simulink model "STEVE_Simulation_6DOF"  (R2025b)
settings: Solver=ode45  StartTime=0  StopTime=60  FixedStep=0.0001  MaxStep=0.0001  RelTol=1e-3
model workspace (MAT data in the model file):
  op_trim1 : opcond.OperatingReport (value not decoded)
undefined symbols (not defined in the file): Actuators, AeroData, C_inner_maxQ_d_Ki, C_inner_maxQ_d_Kp, C_outer_maxQ_d_Ki, C_outer_maxQ_d_Kp, F, launchpad_alt, Light, MIL, PrelookupData, Ref_Area, rocket_length, timeStep, Ts_inner, Ts_outer, warm_up_time, wn_ramp
libraries: simulink_extras x23, simulink x7, slpidlib x5, aerolibwind2 x3, aerolibconvert2 x3, aerolibasang x2, aerolibactuator x2, aerolibatmos2 x1
(part 2 of 2)

== system STEVE_Simulation_6DOF/STeVe System Model/Subsystem/Classical Upgraded/Cascade PID Controller1 ==
  pitch rate : Inport
  pitch : Inport  Port=2
  pitch_setpoint : Inport  Port=3
  Add : Sum  Inputs=-+
  Add1 : Sum  Inputs=-+
  Pitch Controller : slpidlib/PID Controller  Controller=PI  Form=Parallel  TimeDomain=Discrete-time  UseExternalTs=off  SampleTime=Ts_outer  IntegratorMethod=Forward Euler  FilterMethod=Forward Euler  ControllerParametersSource=internal  P=C_outer_maxQ_d_Kp  I=C_outer_maxQ_d_Ki  UseKiTs=off  D=0.164283893804061  UseExternalDerivativeSource=off  N=4651.32243718652  UseFilter=on  TunerSelectOption=Transfer Function Based (PID Tuner App)  InitialConditionSource=internal  InitialConditionForIntegrator=0  InitialConditionForFilter=0  DifferentiatorICPrevScaledInput=0  ExternalReset=none  TrackingMode=off  Kt=1  LimitOutput=off  SatLimitsSource=internal  UpperSaturationLimit=inf  LowerSaturationLimit=-inf  LinearizeAsGain=on  AntiWindupMode=none  Kb=1  LimitIntegrator=off  UpperIntegratorSaturationLimit=inf  LowerIntegratorSaturationLimit=-inf  POutMin=[]  POutMax=[]  IOutMin=[]  IOutMax=[]  DOutMin=[]  DOutMax=[]  NOutMin=[]  NOutMax=[]  SumOutMin=[]  SumOutMax=[]  SaturationOutMin=[]  SaturationOutMax=[]  PParamMin=[]  PParamMax=[]  IParamMin=[]  IParamMax=[]  DParamMin=[]  DParamMax=[]  NParamMin=[]  NParamMax=[]  KbParamMin=[]  KbParamMax=[]  KtParamMin=[]  KtParamMax=[]  KbOutMin=[]  KbOutMax=[]  KtOutMin=[]  KtOutMax=[]  IntegratorOutMin=[]  IntegratorOutMax=[]  FilterOutMin=[]  FilterOutMax=[]  SumI1OutMin=[]  SumI1OutMax=[]  SumI2OutMin=[]  SumI2OutMax=[]  SumI3OutMin=[]  SumI3OutMax=[]  SumI4OutMin=[]  SumI4OutMax=[]  SumDOutMin=[]  SumDOutMax=[]  DifferentiatorOutMin=[]  DifferentiatorOutMax=[]  FilterDiffOutCoefMin=[]  FilterDiffOutCoefMax=[]  ReciprocalOutMin=[]  ReciprocalOutMax=[]  SumDenOutMin=[]  SumDenOutMax=[]  SumNumOutMin=[]  SumNumOutMax=[]  DivideOutMin=[]  DivideOutMax=[]  UdiffTsProdOutMin=[]  UdiffTsProdOutMax=[]  NTsProdOutMin=[]  NTsProdOutMax=[]  UintegralTsProdOutMin=[]  UintegralTsProdOutMax=[]  UngainTsProdOutMin=[]  UngainTsProdOutMax=[]  ClampingZeroOutDataTypeStr=Inherit: Inherit via back propagation  ClampingZeroOutMin=[]  ClampingZeroOutMax=[]  FilterDenConstantOutDataTypeStr=Inherit: Inherit via back propagation  FilterDenConstantOutMin=[]  FilterDenConstantOutMax=[]  PCopyOutDataTypeStr=Inherit: Inherit via back propagation  PCopyOutMin=[]  PCopyOutMax=[]  NCopyOutDataTypeStr=Inherit: Inherit via back propagation  NCopyOutMin=[]  NCopyOutMax=[]  IntegratorContinuousStateAttributes=''  IntegratorStateMustResolveToSignalObject=off  IntegratorRTWStateStorageClass=Auto  FilterContinuousStateAttributes=''  FilterStateMustResolveToSignalObject=off  FilterRTWStateStorageClass=Auto  ParallelPVariant=InternalParameters  IdealPVariant=Disabled  IVariant=InternalParameters  DVariant=Disabled  IntegratorVariant=Discrete  SatVariant=Disabled  AWVariant=Passthrough  PCopyVariant=Disabled  TRVariant=Disabled  FdbkBlocksVariant=Forward  IdealPFdbkVariant=Disabled  SatFdbkVariant=Disabled  DerivativeFilterVariant=Disabled  NVariant=Disabled  NCopyVariant=Disabled_SignalSpec  FilterICVariant=Disabled  IntegratorICVariant=InternalICs  ExternalResetVariant=Disabled  TRSumVariant=Passthrough  SumFdbkVariant=Disabled  SumVariant=Sum_PI  TsampFilterVariant=InternalTs  TsampNgainVariant=Passthrough  TsampIntegralVariant=Disabled_SignalSpec  ExternalSaturationOutDataTypeStr=Inherit: Same as second input  DerivativeSourceVariant=Disabled  PreIntVariant=InternalPreInt
  Pitch Rate Controller : slpidlib/PID Controller  Controller=PI  Form=Parallel  TimeDomain=Discrete-time  UseExternalTs=off  SampleTime=Ts_inner  IntegratorMethod=Forward Euler  FilterMethod=Forward Euler  ControllerParametersSource=internal  P=C_inner_maxQ_d_Kp  I=C_inner_maxQ_d_Ki  UseKiTs=off  D=0.164283893804061  UseExternalDerivativeSource=off  N=4651.32243718652  UseFilter=on  TunerSelectOption=Transfer Function Based (PID Tuner App)  InitialConditionSource=internal  InitialConditionForIntegrator=0  InitialConditionForFilter=0  DifferentiatorICPrevScaledInput=0  ExternalReset=none  TrackingMode=off  Kt=1  LimitOutput=off  SatLimitsSource=internal  UpperSaturationLimit=inf  LowerSaturationLimit=-inf  LinearizeAsGain=on  AntiWindupMode=none  Kb=1  LimitIntegrator=off  UpperIntegratorSaturationLimit=inf  LowerIntegratorSaturationLimit=-inf  POutMin=[]  POutMax=[]  IOutMin=[]  IOutMax=[]  DOutMin=[]  DOutMax=[]  NOutMin=[]  NOutMax=[]  SumOutMin=[]  SumOutMax=[]  SaturationOutMin=[]  SaturationOutMax=[]  PParamMin=[]  PParamMax=[]  IParamMin=[]  IParamMax=[]  DParamMin=[]  DParamMax=[]  NParamMin=[]  NParamMax=[]  KbParamMin=[]  KbParamMax=[]  KtParamMin=[]  KtParamMax=[]  KbOutMin=[]  KbOutMax=[]  KtOutMin=[]  KtOutMax=[]  IntegratorOutMin=[]  IntegratorOutMax=[]  FilterOutMin=[]  FilterOutMax=[]  SumI1OutMin=[]  SumI1OutMax=[]  SumI2OutMin=[]  SumI2OutMax=[]  SumI3OutMin=[]  SumI3OutMax=[]  SumI4OutMin=[]  SumI4OutMax=[]  SumDOutMin=[]  SumDOutMax=[]  DifferentiatorOutMin=[]  DifferentiatorOutMax=[]  FilterDiffOutCoefMin=[]  FilterDiffOutCoefMax=[]  ReciprocalOutMin=[]  ReciprocalOutMax=[]  SumDenOutMin=[]  SumDenOutMax=[]  SumNumOutMin=[]  SumNumOutMax=[]  DivideOutMin=[]  DivideOutMax=[]  UdiffTsProdOutMin=[]  UdiffTsProdOutMax=[]  NTsProdOutMin=[]  NTsProdOutMax=[]  UintegralTsProdOutMin=[]  UintegralTsProdOutMax=[]  UngainTsProdOutMin=[]  UngainTsProdOutMax=[]  ClampingZeroOutDataTypeStr=Inherit: Inherit via back propagation  ClampingZeroOutMin=[]  ClampingZeroOutMax=[]  FilterDenConstantOutDataTypeStr=Inherit: Inherit via back propagation  FilterDenConstantOutMin=[]  FilterDenConstantOutMax=[]  PCopyOutDataTypeStr=Inherit: Inherit via back propagation  PCopyOutMin=[]  PCopyOutMax=[]  NCopyOutDataTypeStr=Inherit: Inherit via back propagation  NCopyOutMin=[]  NCopyOutMax=[]  IntegratorContinuousStateAttributes=''  IntegratorStateMustResolveToSignalObject=off  IntegratorRTWStateStorageClass=Auto  FilterContinuousStateAttributes=''  FilterStateMustResolveToSignalObject=off  FilterRTWStateStorageClass=Auto  ParallelPVariant=InternalParameters  IdealPVariant=Disabled  IVariant=InternalParameters  DVariant=Disabled  IntegratorVariant=Discrete  SatVariant=Disabled  AWVariant=Passthrough  PCopyVariant=Disabled  TRVariant=Disabled  FdbkBlocksVariant=Forward  IdealPFdbkVariant=Disabled  SatFdbkVariant=Disabled  DerivativeFilterVariant=Disabled  NVariant=Disabled  NCopyVariant=Disabled_SignalSpec  FilterICVariant=Disabled  IntegratorICVariant=InternalICs  ExternalResetVariant=Disabled  TRSumVariant=Passthrough  SumFdbkVariant=Disabled  SumVariant=Sum_PI  TsampFilterVariant=InternalTs  TsampNgainVariant=Passthrough  TsampIntegralVariant=Disabled_SignalSpec  ExternalSaturationOutDataTypeStr=Inherit: Same as second input  DerivativeSourceVariant=Disabled  PreIntVariant=InternalPreInt
  nozzle angle : Outport
  wires:
  pitch/1 -> Add/1
  pitch_setpoint/1 -> Add/2
  Add/1 -> Pitch Controller/1
  Add1/1 -> Pitch Rate Controller/1
  pitch rate/1 -> Add1/1
  Pitch Controller/1 -> Add1/2
  Pitch Rate Controller/1 -> nozzle angle/1

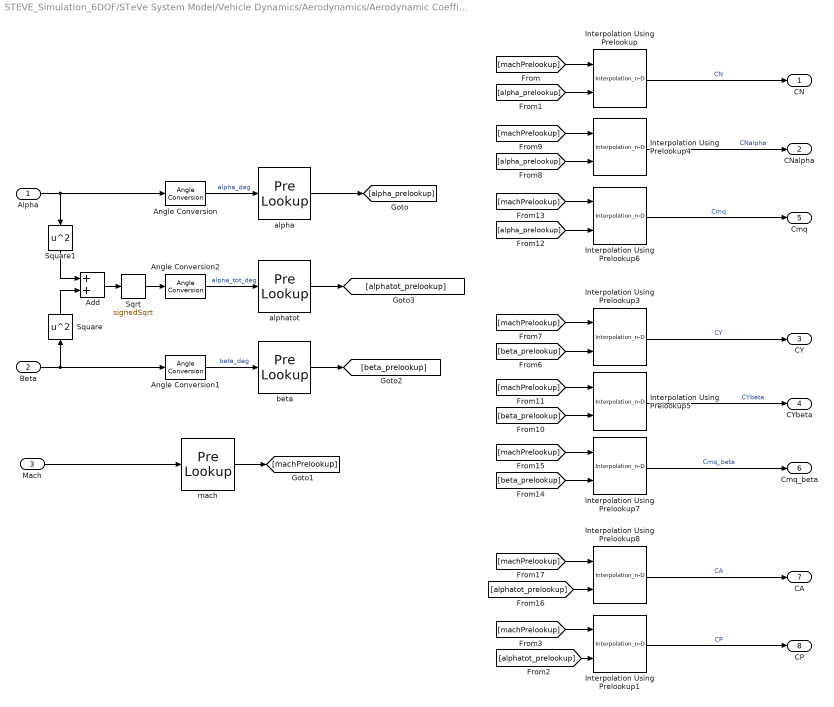
== system STEVE_Simulation_6DOF/STeVe System Model/Vehicle Dynamics/Aerodynamics/Aerodynamic Coefficients  ==
  Alpha : Inport
  Beta : Inport  Port=2
  Mach : Inport  Port=3
  Add : Sum
  Angle Conversion : aerolibconvert2/Angle Conversion  IU=rad  OU=deg
  Angle Conversion1 : aerolibconvert2/Angle Conversion  IU=rad  OU=deg
  Angle Conversion2 : aerolibconvert2/Angle Conversion  IU=rad  OU=deg
  Interpolation Using Prelookup : Interpolation_n-D  Table=AeroData.Tables.CN  RequireIndexFractionAsBus=on  InternalRulePriority=Speed
      settings: InputPortMap=u0,u1
  Interpolation Using Prelookup1 : Interpolation_n-D  Table=AeroData.Tables.CP  RequireIndexFractionAsBus=on  InternalRulePriority=Speed
      settings: InputPortMap=u0,u1
  Interpolation Using Prelookup3 : Interpolation_n-D  Table=AeroData.Tables.CY  RequireIndexFractionAsBus=on  InternalRulePriority=Speed
      settings: InputPortMap=u0,u1
  Interpolation Using Prelookup4 : Interpolation_n-D  Table=AeroData.Tables.CNalpha  RequireIndexFractionAsBus=on  InternalRulePriority=Speed
      settings: InputPortMap=u0,u1
  Interpolation Using Prelookup5 : Interpolation_n-D  Table=AeroData.Tables.CYbeta  RequireIndexFractionAsBus=on  InternalRulePriority=Speed
      settings: InputPortMap=u0,u1
  Interpolation Using Prelookup6 : Interpolation_n-D  Table=AeroData.Tables.Cmq  RequireIndexFractionAsBus=on  InternalRulePriority=Speed
      settings: InputPortMap=u0,u1
  Interpolation Using Prelookup7 : Interpolation_n-D  Table=AeroData.Tables.Cmq_beta  RequireIndexFractionAsBus=on  InternalRulePriority=Speed
      settings: InputPortMap=u0,u1
  Interpolation Using Prelookup8 : Interpolation_n-D  Table=AeroData.Tables.CA  RequireIndexFractionAsBus=on  InternalRulePriority=Speed
      settings: InputPortMap=u0,u1
  Sqrt : Sqrt  Operator=signedSqrt
  Square : Math  Operator=square
  Square1 : Math  Operator=square
  alpha : PreLookup  BreakpointsData=AeroData.Breakpoints.Alpha  OutputSelection=Index and fraction as bus  IndexSearchMethod=Evenly spaced points  UseLastBreakpoint=on
  alphatot : PreLookup  BreakpointsData=AeroData.Breakpoints.AlphaTot  OutputSelection=Index and fraction as bus  IndexSearchMethod=Evenly spaced points  UseLastBreakpoint=on
  beta : PreLookup  BreakpointsData=AeroData.Breakpoints.Beta  OutputSelection=Index and fraction as bus  IndexSearchMethod=Evenly spaced points  UseLastBreakpoint=on
  mach : PreLookup  BreakpointsData=AeroData.Breakpoints.Mach  OutputSelection=Index and fraction as bus  IndexSearchMethod=Evenly spaced points  ExtrapMethod=Linear
  CN : Outport
  CNalpha : Outport  Port=2
  CY : Outport  Port=3
  CYbeta : Outport  Port=4
  Cmq : Outport  Port=5
  Cmq_beta : Outport  Port=6
  CA : Outport  Port=7
  CP : Outport  Port=8
  wires:
  Interpolation Using Prelookup/1 -> CN/1  "CN"
  alpha/1 -> [alpha_prelookup]
  mach/1 -> [machPrelookup]
  [machPrelookup] -> Interpolation Using Prelookup/1
  [alpha_prelookup] -> Interpolation Using Prelookup/2
  Angle Conversion/1 -> alpha/1  "alpha_deg"
  Mach/1 -> mach/1
  Alpha/1 -> Square1/1, Angle Conversion/1
  Beta/1 -> Square/1, Angle Conversion1/1
  Angle Conversion1/1 -> beta/1  "beta_deg"
  beta/1 -> [beta_prelookup]
  Add/1 -> Sqrt/1
  Square1/1 -> Add/1
  Square/1 -> Add/2
  alphatot/1 -> [alphatot_prelookup]
  Angle Conversion2/1 -> alphatot/1  "alpha_tot_deg"
  Sqrt/1 -> Angle Conversion2/1
  [alpha_prelookup] -> Interpolation Using Prelookup4/2
  [machPrelookup] -> Interpolation Using Prelookup4/1
  Interpolation Using Prelookup4/1 -> CNalpha/1  "CNalpha"
  [machPrelookup] -> Interpolation Using Prelookup3/1
  [beta_prelookup] -> Interpolation Using Prelookup3/2
  Interpolation Using Prelookup3/1 -> CY/1  "CY"
  [machPrelookup] -> Interpolation Using Prelookup5/1
  Interpolation Using Prelookup5/1 -> CYbeta/1  "CYbeta"
  [beta_prelookup] -> Interpolation Using Prelookup5/2
  [machPrelookup] -> Interpolation Using Prelookup6/1
  [alpha_prelookup] -> Interpolation Using Prelookup6/2
  Interpolation Using Prelookup6/1 -> Cmq/1  "Cmq"
  [machPrelookup] -> Interpolation Using Prelookup7/1
  Interpolation Using Prelookup7/1 -> Cmq_beta/1  "Cmq_beta"
  [beta_prelookup] -> Interpolation Using Prelookup7/2
  [machPrelookup] -> Interpolation Using Prelookup8/1
  Interpolation Using Prelookup8/1 -> CA/1  "CA"
  [alphatot_prelookup] -> Interpolation Using Prelookup8/2
  Interpolation Using Prelookup1/1 -> CP/1  "CP"
  [alphatot_prelookup] -> Interpolation Using Prelookup1/2
  [machPrelookup] -> Interpolation Using Prelookup1/1

== system STEVE_Simulation_6DOF/STeVe System Model/Vehicle Dynamics/Aerodynamics/DerivedConditions ==
  Speed of sound : Inport
  Air Density : Inport  Port=2
  uvw_b_w : Inport  Port=3
  Dynamic Pressure : aerolibasang/Dynamic Pressure
  MATLAB Function : MATLAB Function  TreatAsAtomicUnit=on
  Mach Number : aerolibasang/Mach Number  Commented=on
  Mach : Outport
  qbar : Outport  Port=2
  wires:
  Speed of sound/1 -> MATLAB Function/2(a)
  uvw_b_w/1 -> MATLAB Function/1(uvw), Dynamic Pressure/1
  MATLAB Function/1(M) -> Mach/1  "Mach"
  Air Density/1 -> Dynamic Pressure/2
  Dynamic Pressure/1 -> qbar/1  "qbar"

== system STEVE_Simulation_6DOF/STeVe System Model/Vehicle Dynamics/Time Varying Parameters/TimeToIndex ==
  t : Inport
  Add Constant : Bias  Bias=1  SaturateOnIntegerOverflow=off
  Constant : Constant  Value=timeStep
  Product : Product  Inputs=*/
  Index : Outport
  wires:
  t/1 -> Product/1
  Constant/1 -> Product/2
  Product/1 -> Add Constant/1
  Add Constant/1 -> Index/1

== matlab function STEVE_Simulation_6DOF/STeVe System Model/Vehicle Dynamics/RocketEngineActuators/MATLAB Function ==
  data: altitude input; thrust output
function thrust = fcn(altitude)

thrust = -3.75507*10^(-2)*altitude + 2.76476*10^(4);

== matlab function STEVE_Simulation_6DOF/Environment/g(h) ==
  data: h input; g output
function g = fcn(h)
G = 6.67430*10^(-11);
M = 5.9722*10^(24);
R_e = 6.371*10^(6);

g = (G * M)/(R_e + h)^2;

== matlab function STEVE_Simulation_6DOF/STeVe System Model/Vehicle Dynamics/Aerodynamics/MATLAB Function ==
  data: CN input; F_b output; CNalpha input; CY input; CYbeta input; Cmq input; Cmq_beta input; CA input; CP_from_nose input; Ref_Area input; CG_from_nose input; omega_pqr input; airspeed input; ref_length input; air_density input; M_b output
function [F_b, M_b] = aero_forces_moments( ...
    CN, CNalpha, CY, CYbeta, Cmq, Cmq_beta, CA, CP_from_nose, ...
    Ref_Area, CG_from_nose, omega_pqr, airspeed, ref_length, air_density)
% Aero forces and moments (body axes), with beta convention:
%   Positive beta = wind from the right
% Inputs:
%   CN, CY, CA             : force coefficients
%   CNalpha, CYbeta        : slopes (reserved)
%   Cmq, Cmq_beta          : damping (pitch/yaw), lumped
%   CP_from_nose, CG_from_nose : [m]
%   Ref_Area               : [m^2]
%   ref_length             : [m]
%   omega_pqr              : [rad/s] [p; q; r]
%   airspeed               : [m/s]
%   air_density            : [kg/m^3]
% Outputs:
%   F_b = [Fx; Fy; Fz], M_b = [Mx; My; Mz]



% --- Precompute
S  = Ref_Area;
d  = ref_length;
V  = max(airspeed, 1e-6);
q_dyn = 0.5 * air_density * V * V;
Lcp = CP_from_nose - CG_from_nose;

% Body rates
p = omega_pqr(1);
q = omega_pqr(2);
r = omega_pqr(3);

% --- Adjust lateral force for beta sign convention (positive beta = wind from right)
CY_eff = -CY;

% --- Forces (x forward, y right, z down)
Fx = - q_dyn * S * CA;
Fy =   q_dyn * S * CY_eff;
Fz = - q_dyn * S * CN;

% --- Static moments from CP lever arm
M_stat_x = 0.0;
M_stat_y = - q_dyn * S * CN     * Lcp;
M_stat_z = - q_dyn * S * CY_eff * Lcp;

% --- Rate damping with d/(2V) (Cmq and Cmq_beta are negative for damping, keep as-is)
scale = d / (2.0 * V);
M_damp_y = q_dyn * S * d * ( scale * Cmq      * q );
M_damp_z = q_dyn * S * d * ( scale * Cmq_beta * r );

% --- Totals
Mx = M_stat_x;
My = M_stat_y + M_damp_y;
Mz = M_stat_z + M_damp_z;

F_b = [Fx; Fy; Fz];
M_b = [Mx; My; Mz];
end

== matlab function STEVE_Simulation_6DOF/STeVe System Model/Vehicle Dynamics/6DOF Equations of Motion/MATLAB Function ==
  data: v_E input; alpha output; R_BE input; wind_uvw input; beta output; alpha_total output; V_air output; uvw_b output
function [alpha, beta, alpha_total, V_air, uvw_b] = aero_angles(v_E, R_BE, wind_uvw)
% Aerodynamic angles from Earth velocity, quaternion (Earth->Body), and wind.
% Convention: positive beta = wind from the RIGHT (opposite thesis sign)
% Units: radians, m/s

% -- Parameters
VEL_EPS = 1e-6;

% -- Relative air-velocity in body axes
v_b = R_BE * v_E(:);
uvw_b = v_b - wind_uvw(:);

u = uvw_b(1); v = uvw_b(2); w = uvw_b(3);
V_air = norm(uvw_b);

% -- Handle zero/near-zero airspeed
if V_air < VEL_EPS
    alpha = 0.0;
    beta  = 0.0;
    alpha_total = 0.0;
    uvw_b = [0;0;0];
    V_air = 0.0;
    return
end

% -- Aerodynamic angles (robust)
alpha = atan2(w, u);
beta  = asin( max(-1, min(1, v / V_air)) );
alpha_total = sqrt(alpha^2 + beta^2);

end

== matlab function STEVE_Simulation_6DOF/STeVe System Model/Vehicle Dynamics/Propulsion F,M/MATLAB Function ==
  data: pitch_angle_rad input; F_body output; yaw_angle_rad input; engine_thrust input; L_cg input; M_body output
function [F_body, M_body] = calculate_tvc_forces_moments(pitch_angle_rad, yaw_angle_rad, engine_thrust, L_cg)
    % Calculates the forces and moments generated by a thrust-vectoring nozzle.
    %
    % Coordinate System:
    % X-axis: along rocket body (forward/out the nose)
    % Y-axis: lateral (starboard/right)
    % Z-axis: normal (down)
    %
    % Angle Conventions (Right-Hand Rule):
    % pitch_angle_rad: Positive rotation about the Y-axis (deflects nozzle down, creates F_z force)
    % yaw_angle_rad:   Positive rotation about the Z-axis (deflects nozzle right, creates F_y force)

    % Decompose thrust into body-frame force components
    % This decomposition assumes a Z-Y rotation sequence (yaw then pitch)
    F_x = engine_thrust * cos(pitch_angle_rad) * cos(yaw_angle_rad);
    F_y = engine_thrust * sin(yaw_angle_rad);
    F_z = engine_thrust * cos(yaw_angle_rad) * sin(pitch_angle_rad);
    
    % Body forces vector [N]
    F_body = [F_x; F_y; F_z];
    
    % Calculate moments about the Center of Gravity (CG)
    % Moment arm from CG to nozzle is r = [-L_cg, 0, 0]
    % Moment M = r x F
    
    % Roll moment (about x-axis) - typically zero for a single nozzle
    M_roll = 0;
    
    % Pitch moment (about y-axis)
    M_pitch = L_cg * F_z;
    
    % Yaw moment (about z-axis)
    M_yaw = L_cg * F_y;
    
    % Body moments vector [N*m]
    M_body = [M_roll; M_pitch; M_yaw];
end

== matlab function STEVE_Simulation_6DOF/STeVe System Model/Vehicle Dynamics/Aerodynamics/DerivedConditions/MATLAB Function ==
  data: uvw input; M output; a input
function M = mach_from_uvw(uvw, a)
% MACH_FROM_UVW  Mach number from body-axes wind [u v w] and speed of sound.
%   M = mach_from_uvw(uvw, a)
%   - uvw: [N x 3] or [3 x N] array of velocities (m/s), negative components allowed
%   - a  : scalar or vector speed of sound (m/s)
% Returns:
%   - M  : Mach number, size matches number of samples in uvw

% --- Input parsing
validateattributes(uvw, {'numeric'}, {'nonempty','real','finite'});
validateattributes(a,   {'numeric'}, {'nonempty','real','finite'});

% --- Velocity magnitude (handles negative components)
if size(uvw,2) == 3
    vmag = vecnorm(uvw, 2, 2);     % N x 1
elseif size(uvw,1) == 3
    vmag = vecnorm(uvw, 2, 1).';   % N x 1
else
    error('uvw must be N-by-3 or 3-by-N.');
end

% --- Speed of sound handling (ensure positive and nonzero)
a = abs(a);                        % Mach uses positive local sound speed
if isscalar(a)
    a = repmat(max(a, eps), size(vmag));
else
    a = a(:);
    if numel(a) ~= numel(vmag)
        error('Length of a must match number of samples in uvw or be scalar.');
    end
    a = max(a, eps);               % avoid divide-by-zero
end

% --- Mach number
M = vmag ./ a;
end

== matlab function STEVE_Simulation_6DOF/STeVe System Model/Vehicle Dynamics/Aerodynamics/MATLAB Function1 ==
  data: qbar input; S input; xcp_from_nose input; xcg_from_nose input; CNa input; dMdalpha output
function dMdalpha = dMdalpha_simple(qbar, S, xcp_from_nose, xcg_from_nose, CNa)
% --- Aero pitching-moment derivative about CG [N*m/rad]
% Inputs (SI): qbar [N/m^2], S [m^2], xcp_from_nose [m], xcg_from_nose [m], CNa [1/rad]
% Coordinates: x measured from nose toward tail

% lever arm CP minus CG
lever = xcg_from_nose - xcp_from_nose;

% small-angle aero moment derivative
dMdalpha = qbar * S * lever * CNa;
end

== matlab function STEVE_Simulation_6DOF/STeVe System Model/Vehicle Dynamics/Aerodynamics/MATLAB Function2 ==
  data: qbar input; S input; Lref input; V input; Cmq input; Mq output
function Mq = dMdq_simple(qbar, S, Lref, V, Cmq)
% --- Aero pitch-rate damping derivative M_q [N*m/(rad/s)]
% Inputs (SI):
%   qbar : dynamic pressure [N/m^2]
%   S    : reference area [m^2]
%   Lref : reference length (e.g., diameter/chord) [m]
%   V    : true airspeed [m/s]
%   Cmq  : pitching-moment coefficient derivative wrt pitch rate (dimensionless)
%
% Output:
%   Mq   : dM/dq [N*m/(rad/s)]

Mq = qbar * S * (Lref^2 / (2*max(V, eps))) * Cmq;
end
